simulink model "TUNABLE_BLOCK"  (R2024b)
settings: Solver=VariableStepAuto  StartTime=0.0  StopTime=10.0  RelTol=1e-3
settings Model: Creator=415  LastModifiedBy=415

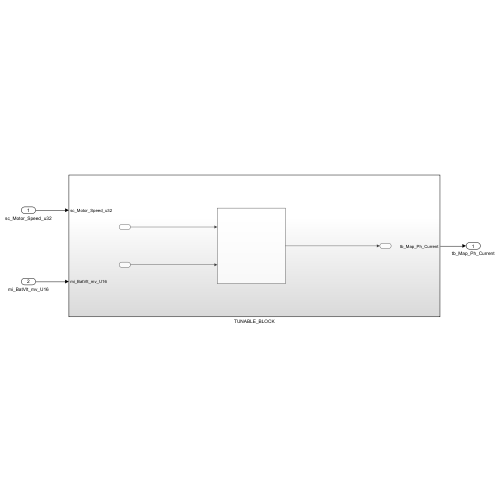
[thumbnail: Simulink's stored preview of the top-level diagram]
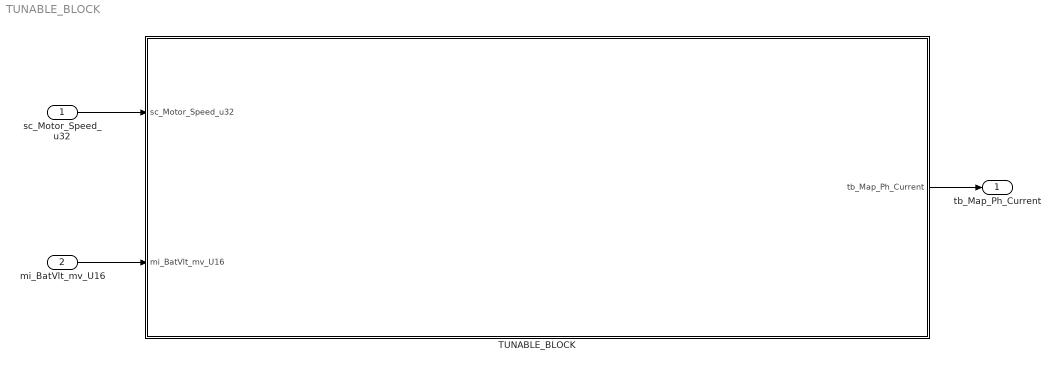
== system TUNABLE_BLOCK ==
  sc_Motor_Speed_u32 : Inport
  mi_BatVlt_mv_U16 : Inport  Port=2
  TUNABLE_BLOCK : Subsystem
  tb_Map_Ph_Current : Outport
  wires:
  sc_Motor_Speed_u32/1 -> TUNABLE_BLOCK/1(sc_Motor_Speed_u32)
  mi_BatVlt_mv_U16/1 -> TUNABLE_BLOCK/2(mi_BatVlt_mv_U16)
  TUNABLE_BLOCK/1(tb_Map_Ph_Current) -> tb_Map_Ph_Current/1

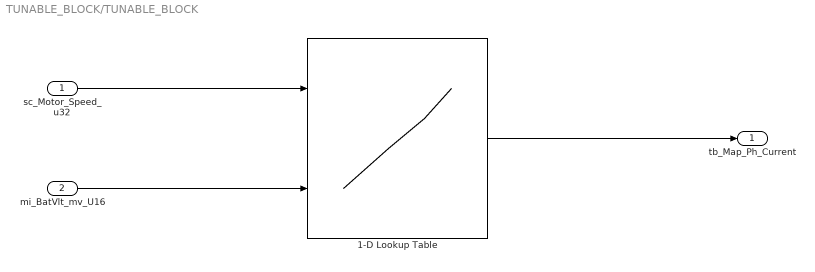
== system TUNABLE_BLOCK/TUNABLE_BLOCK ==
  sc_Motor_Speed_u32 : Inport
  mi_BatVlt_mv_U16 : Inport  Port=2
  1-D Lookup Table : Lookup_n-D  BreakpointsForDimension1=[0;1000;2000;3000;4000;5000;6000;7000;8000;9000;10000;11000;12000;13000;14000;15000;16000;17000;18000;19000;20000;21000;22000;23000;24000;25000]  BreakpointsForDimension2=[29000;30000;31000;32000;33000;34000;35000;36000;37000;38000;39000;40000;41000;42000]  Table=[9700 10000 14500 20800 28800 36000 36000 36000 36000 36000 36000 36000 36000 36000;8000 8400 12800 19000 27000 36000 36000 36000 36000 36000 36000 36000 36000 36000;6800 7200 11200 17400 25400 36000 36000 36000 36000 36000 36000 36000 36000 36000;5800 6000 10000 15800 23800 36000 36000 36000 36000 36000 36000 36000 36000 36000;4900 5100 8800 14500 22400 34600 35200 35800 36000 36000 36000 36000 36000 36000;4300 4400 8000 13400 21000 33100 33700 34300 34800 35400 36000 36000 36000 36000;3700 3900 7000 12400 19800 31700 32300 32900 33500 34000 34600 35100 35700 36000;3300 3400 6400 11500 18700 30400 31000 31600 32100 32700 33200 33800 34300 34800;3000 3100 6000 10700 17600 29200 29700 30300 30800 31400 31900 32500 33000 33500;2700 2800 5500 9900 16700 28000 28500 29100 29600 30200 30700 31200 31800 32200;2500 2600 5000 9300 15800 26800 27400 27900 28500 29000 29500 30100 30600 31100;2300 2300 4600 8700 15000 25800 26300 26900 27400 27900 28400 28900 29500 29900;2100 2200 4300 8200 14200 24800 25300 25800 26400 26900 27400 27900 28400 28900;1900 2000 4000 7700 13500 23800 24400 24900 25400 25900 26400 26900 27400 27800;1800 1900 3800 7300 12900 22900 23500 24000 24500 25000 25500 25900 26400 26900;1700 1800 3500 6900 12300 22100 22600 23100 23600 24100 24600 25000 25500 26000;1600 1700 3300 6500 11700 21300 21800 22300 22800 23200 23700 24200 24700 25100;1500 1600 3200 6200 11200 20600 21000 21500 22000 22500 22900 23400 23800 24300;1400 1500 3000 5900 10800 19800 20300 20800 21200 21700 22200 22600 23100 23500;1400 1400 2900 5700 10300 19200 19600 20100 20500 21000 21400 21900 22300 22700;1300 1300 2700 5400 9900 18500 19000 19400 19900 20300 20800 21200 21600 22000;1200 1300 2600 5200 9600 17900 18400 18800 19300 19700 20100 20500 21000 21400;1200 1200 2500 5000 9200 17400 17800 18200 18700 19100 19500 19900 20300 20700;1100 1200 2400 4800 8900 16800 17300 17700 18100 18500 18900 19300 19700 20100;1100 1100 2300 4600 8600 16300 16700 17100 17600 18000 18400 18800 19200 19600;1000 1100 2200 4400 8300 15800 16200 16600 17000 17400 17800 18200 18600 19000]  InternalRulePriority=Speed  RndMeth=Simplest
      settings: InputPortMap=u0,u1
  tb_Map_Ph_Current : Outport
  wires:
  1-D Lookup Table/1 -> tb_Map_Ph_Current/1
  sc_Motor_Speed_u32/1 -> 1-D Lookup Table/1
  mi_BatVlt_mv_U16/1 -> 1-D Lookup Table/2
